simulink model "BPSK_TX_Nishat"  (R2018a)
settings: Solver=VariableStepAuto  StartTime=0.0  StopTime=inf  RelTol=1e-3
values from neighbouring files (symbols this model uses):
  BitRate = 100    [BitRate.mat]
undefined symbols (not defined in the file or in its folder): gcbh, rcfiltgaincompat
libraries: commdigbbndpm3 x2, simulink x2, commfilt2 x2, commsdrhw_v2 x2, commrandsrc2 x1, commseqgen3 x1
settings Model: Creator=n53s123  LastModifiedBy=n53s123

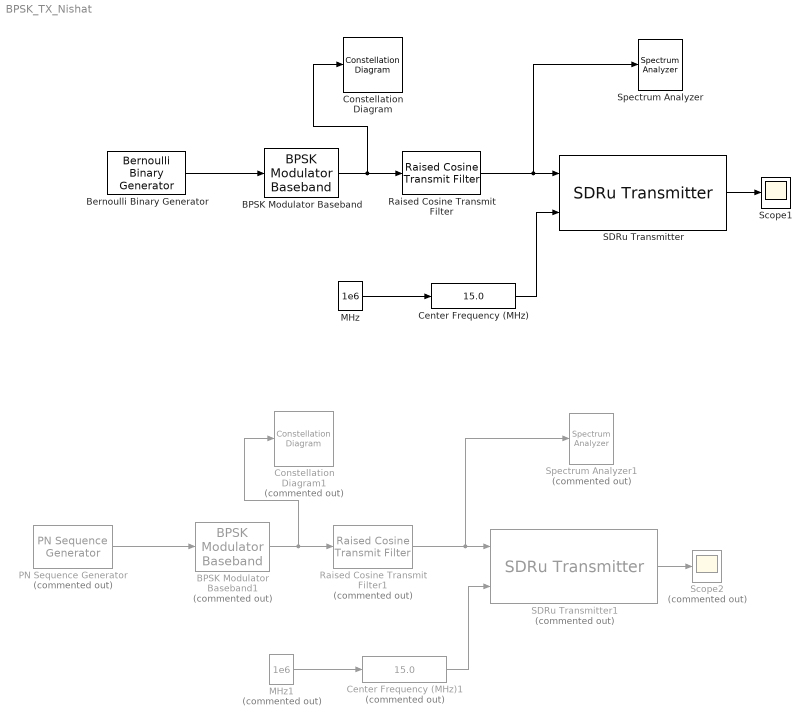
== system BPSK_TX_Nishat ==
  BPSK Modulator Baseband : commdigbbndpm3/BPSK Modulator Baseband  Ph=0  outDtype=double  outWordLen=16  outUDDataType=sfix(16)  outFracLenMode=Best precision  outFracLen=15  outDataTypeStr=double  outLastDataTypeStr=double
  BPSK Modulator Baseband1 : commdigbbndpm3/BPSK Modulator Baseband  Commented=on  Ph=0  outDtype=double  outWordLen=16  outUDDataType=sfix(16)  outFracLenMode=Best precision  outFracLen=15  outDataTypeStr=double  outLastDataTypeStr=double
  Bernoulli Binary Generator : commrandsrc2/Bernoulli Binary Generator  P=0.5  seed=61  Ts=1/BitRate*1000  frameBased=on  sampPerFrame=1000  orient=off  outDataType=boolean
  Center Frequency (MHz) : simulink/Math Operations/Slider Gain  gain=15.0  low=0  high=30
  Center Frequency (MHz)1 : simulink/Math Operations/Slider Gain  Commented=on  gain=15.0  low=0  high=30
  Constellation Diagram : ConstellationDiagram
  Constellation Diagram1 : ConstellationDiagram  Commented=on
  MHz : Constant  Value=1e6  FramePeriod=-1
  MHz1 : Constant  Commented=on  Value=1e6  FramePeriod=-1
  PN Sequence Generator : commseqgen3/PN Sequence Generator  Commented=on  poly='z^6 + z + 1'  ini_sta=[0 0 0 0 0 1]  outBitMaskSource=Dialog parameter  shift=0  outVarSiz=off  maxOutSizeMode=Dialog parameter  maxOutSize=[10 1]  Ts=1/BitRate*4000  sampPerFrame=4000  reset=off  bitPackedOutputs=off  outDataType=double  numPackedBits=8  bitPackDataSigned=off  bitPackedOutDType=double
      settings: SourceProductName=Communications System Toolbox
  Raised Cosine Transmit Filter : commfilt2/Raised Cosine Transmit Filter  filtType=Square root  R=0.5  filtSpan=10  N=2  filterGain=rcfiltgaincompat(gcbh)  InputProcessing=Columns as channels (frame based)  RateOptions=Enforce single-rate processing  framing=Mute  checkCoeff=off  variableName=rcTxFilt  checkGain=Normalized  sampMode=Mute  saveAsFlag=0  currentFiltSpan=2*(5)  D=5  launchFVT=off  roundingMode=Floor  overflowMode=off  coeffDataTypeStr=Inherit: Same word length as input  coeffMin=[]  coeffMax=[]  coeffLastDataTypeStr=Inherit: Same word length as input  outputDataTypeStr=Inherit: Same as accumulator  outputMin=[]  outputMax=[]  outputLastDataTypeStr=Inherit: Same as accumulator
  Raised Cosine Transmit Filter1 : commfilt2/Raised Cosine Transmit Filter  Commented=on  filtType=Square root  R=0.5  filtSpan=2*(5)  N=2  filterGain=rcfiltgaincompat(gcbh)  InputProcessing=Columns as channels (frame based)  RateOptions=Enforce single-rate processing  framing=Mute  checkCoeff=off  variableName=rcTxFilt1  checkGain=Normalized  sampMode=Mute  saveAsFlag=0  currentFiltSpan=2*(5)  D=5  launchFVT=off  roundingMode=Floor  overflowMode=off  coeffDataTypeStr=Inherit: Same word length as input  coeffMin=[]  coeffMax=[]  coeffLastDataTypeStr=Inherit: Same word length as input  outputDataTypeStr=Inherit: Same as accumulator  outputMin=[]  outputMax=[]  outputLastDataTypeStr=Inherit: Same as accumulator
  SDRu Transmitter : commsdrhw_v2/SDRu Transmitter  SourceLibraryInfo="This block requires <a href=\"http://www.mathworks.com/hardware-support/usrp.html\">Communications System Toolbox Support Package for USRP Radio</a>"  rxtx=tx  initializeIPAddress=0  devMap=0  USRP2_IP=192.168.10.2  USRP_IP_X300=192.168.10.2  USRP_IP_X310=192.168.10.2  USRP_serialNumB200=No devices found  USRP_serialNumB210=No devices found  platform=N200/N210/USRP2  prevPlatform=N200/N210/USRP2  lastIPAddressPopup=192.168.10.2  USRP_ID=192.168.10.2  LastIPAddress=192.168.10.2  ChannelMapping=1  centerFrequencySrc=Input port  centerFrequency=2.45e9  loOffsetSrc=Dialog  loOffset=0  gainSrc=Dialog  gain=0  PPSSource=Internal  clockSource=Internal  masterClkRateParam=100e6  masterClkRateB200=32e6  masterClkRateB210=32e6  masterClkRateX300=120e6  masterClkRateX310=120e6  decimInterpSrc=Dialog  decimInterp=512  USRP2_IP_NUM=[49 57 50 46 49 54 56 46 49 48 46 50]  frameLength=362  TransportDataType=int16  outputDatatype=Same as transport data type  overrunUnderrunPort=on  sampleTime=1  dboardInfo=|  HOST_DATA_PORT=30000  HOST_CONTROL_PORT=30001  USRP2_DATA_PORT=32769  USRP2_CONTROL_PORT=32768  bufferMode=Continuous streaming  EnableBurstMode=off  NumFramesInBurst=1
      | dbid: 0
      |           dbName: 'no db found'
      |          freqMin: 0
      |          freqMax: 0
      |          gainMin: 0
      |          gainMax: 0
      |     gainStepSize: 0
      settings: SourceProductName=Communications System Toolbox Support Package for USRP(R) Radio  SourceProductBaseCode=USRP
  SDRu Transmitter1 : commsdrhw_v2/SDRu Transmitter  Commented=on  SourceLibraryInfo="This block requires <a href=\"http://www.mathworks.com/hardware-support/usrp.html\">Communications System Toolbox Support Package for USRP Radio</a>"  rxtx=tx  initializeIPAddress=0  devMap=0  USRP2_IP=192.168.10.2  USRP_IP_X300=192.168.10.2  USRP_IP_X310=192.168.10.2  USRP_serialNumB200=No devices found  USRP_serialNumB210=No devices found  platform=N200/N210/USRP2  prevPlatform=N200/N210/USRP2  lastIPAddressPopup=192.168.10.2  USRP_ID=192.168.10.2  LastIPAddress=192.168.10.2  ChannelMapping=1  centerFrequencySrc=Input port  centerFrequency=2.45e9  loOffsetSrc=Dialog  loOffset=0  gainSrc=Dialog  gain=0  PPSSource=Internal  clockSource=Internal  masterClkRateParam=100e6  masterClkRateB200=32e6  masterClkRateB210=32e6  masterClkRateX300=120e6  masterClkRateX310=120e6  decimInterpSrc=Dialog  decimInterp=500  USRP2_IP_NUM=[49 57 50 46 49 54 56 46 49 48 46 50]  frameLength=362  TransportDataType=int16  outputDatatype=Same as transport data type  overrunUnderrunPort=on  sampleTime=1  dboardInfo=|  HOST_DATA_PORT=30000  HOST_CONTROL_PORT=30001  USRP2_DATA_PORT=32769  USRP2_CONTROL_PORT=32768  bufferMode=Continuous streaming  EnableBurstMode=off  NumFramesInBurst=1
      | dbid: 0
      |           dbName: 'no db found'
      |          freqMin: 0
      |          freqMax: 0
      |          gainMin: 0
      |          gainMax: 0
      |     gainStepSize: 0
      settings: SourceProductName=Communications System Toolbox Support Package for USRP(R) Radio  SourceProductBaseCode=USRP
  Scope1 : Scope
  Scope2 : Scope  Commented=on
  Spectrum Analyzer : SpectrumAnalyzer
  Spectrum Analyzer1 : SpectrumAnalyzer  Commented=on
  wires:
  BPSK Modulator Baseband/1 -> Constellation Diagram/1, Raised Cosine Transmit Filter/1
  Bernoulli Binary Generator/1 -> BPSK Modulator Baseband/1
  Center Frequency (MHz)/1 -> SDRu Transmitter/2
  SDRu Transmitter/1 -> Scope1/1
  MHz/1 -> Center Frequency (MHz)/1
  Raised Cosine Transmit Filter/1 -> Spectrum Analyzer/1, SDRu Transmitter/1
  Raised Cosine Transmit Filter1/1 -> Spectrum Analyzer1/1, SDRu Transmitter1/1
  Center Frequency (MHz)1/1 -> SDRu Transmitter1/2
  BPSK Modulator Baseband1/1 -> Constellation Diagram1/1, Raised Cosine Transmit Filter1/1
  SDRu Transmitter1/1 -> Scope2/1
  MHz1/1 -> Center Frequency (MHz)1/1
  PN Sequence Generator/1 -> BPSK Modulator Baseband1/1
